simulink model "controled_three_phase_rectifier"  (R2023a)
settings: Solver=ode1be  StartTime=0.0  StopTime=sim_time  FixedStep=50e-6  RelTol=1e-3
values from neighbouring files (symbols this model uses):
  alpha1 = 20    [controled_three_phase_rectifier_script.m]
  alpha2 = 50    [controled_three_phase_rectifier_script.m]
  alpha_steptime1 = 0.4    [controled_three_phase_rectifier_script.m]
  alpha_steptime2 = 0.8    [controled_three_phase_rectifier_script.m]
  gridfreq = 50    [controled_three_phase_rectifier_script.m]
  Rload = 1    [controled_three_phase_rectifier_script.m]
  Vgrid = 6000    [controled_three_phase_rectifier_script.m]
undefined symbols (not defined in the file or in its folder): D1, lagging, pulse
libraries: fl_lib x17, ee_lib x10, nesl_utility x9, batteryecm_lib x1, spsPLL3phLib x1, spsPulseGeneratorThyristor6PulseLib x1
settings Model: Creator=citcea  LastModifiedBy=citcea

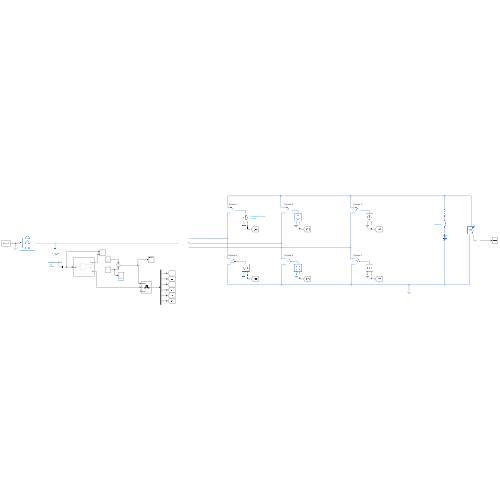
[thumbnail: Simulink's stored preview of the top-level diagram]
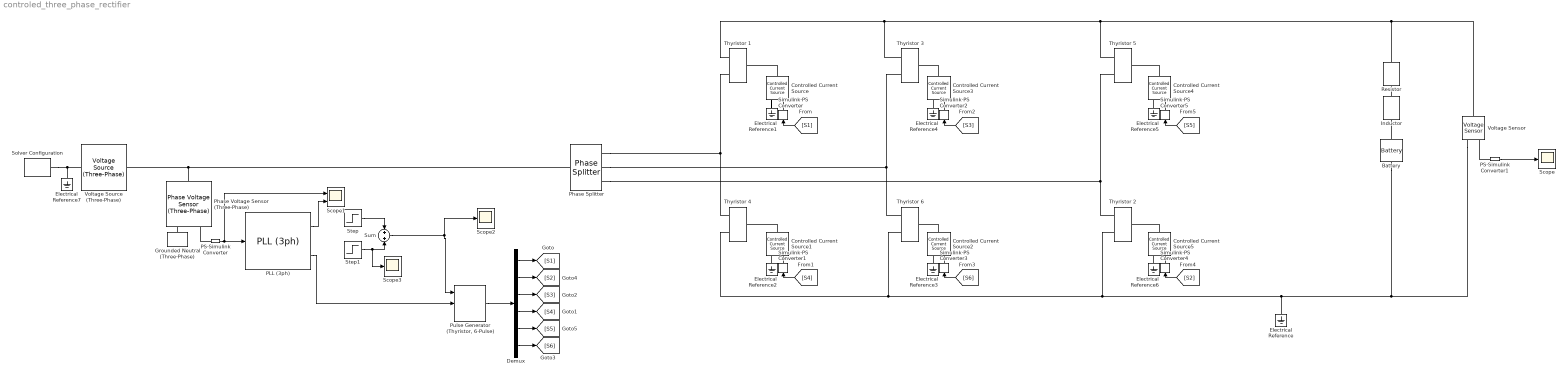
== system controled_three_phase_rectifier ==
  Battery : batteryecm_lib/Battery  Vnom=VDC V  prm_dir=simscape.enum.battery.prm_dir.disabled  R1_dis=2 Ohm  R1_ch=2 Ohm  R1=2 Ohm  prm_AH=simscape.enum.battery.prm_AH.infinite  AH=50 A*hr  V1=11.5 V  AH1=25 A*hr  prm_R2=simscape.enum.battery.prm_R2.disabled  R2=2000 Ohm  Tmeas=298.15 K  charge_measurement_port=simscape.enum.battery.enable.no  prm_dyn=simscape.enum.battery.prm_dyn.off  Rp1=0.005 Ohm  tau1=30 s  Rp2=0.005 Ohm  tau2=30 s  Rp3=0.005 Ohm  tau3=30 s  Rp4=0.005 Ohm  tau4=30 s  Rp5=0.005 Ohm  tau5=30 s  prm_fade=simscape.enum.battery.prm_fade.disabled  N_fade=100  AH_fade=45 A*hr  R1_fade=2.02 Ohm  R1_ch_fade=2.02 Ohm  V1_fade=10.35 V  prm_age=simscape.enum.battery.prm_age.disabled  prm_age_OCV=simscape.enum.battery.prm_age_OCV.OCV  OCV_age=0.9  SOC_age=60  Tmeas_age=298.15 K  delta_time_age_vec=[0] d  temperature_age_vec=[273] K  OCV_scaling_age=2.2134e6  OCV_offset_age=1.632e6  temp_exp_age=0.515833569 V  t_exp_age=0.75  Vnom_T2=12 V  R1_T2=2.2 Ohm  R1_T2_dis=2.2 Ohm  R1_T2_ch=2.2 Ohm  V1_T2=11.4 V  R2_T2=2200 Ohm  Rp1_T2=0.005 Ohm  tau1_T2=30 s  Rp2_T2=0.005 Ohm  tau2_T2=30 s  Rp3_T2=0.005 Ohm  tau3_T2=30 s  Rp4_T2=0.005 Ohm  tau4_T2=30 s  Rp5_T2=0.005 Ohm  tau5_T2=30 s  Tmeas2=273.15 K  thermal_port=simscape.enum.thermaleffects.omit  thermal_mass=30000 J/K  i_specify=off  i_priority=None  i=0 A  i_nominal_specify=off  i_nominal_unit=A  i_nominal_value=1  v_specify=off  v_priority=None  v=0 V  v_nominal_specify=off  v_nominal_unit=V  v_nominal_value=1  charge_specify=off  charge_priority=High  charge=50 A*hr  charge_nominal_specify=off  charge_nominal_unit=A*hr  charge_nominal_value=1  num_cycles_specify=off  num_cycles_priority=High  num_cycles=0  num_cycles_nominal_specify=off  num_cycles_nominal_unit=1  num_cycles_nominal_value=1  temperature_specify=off  temperature_priority=High  temperature=298.15 K  temperature_nominal_specify=off  temperature_nominal_unit=K  temperature_nominal_value=1
  Controlled Current Source{,1..5} (6 alike) : fl_lib/Electrical/Electrical Sources/Controlled Current Source
  Demux : Demux  Outputs=6
  Electrical Reference{,1..7} (8 alike) : fl_lib/Electrical/Electrical Elements/Electrical Reference
  Grounded Neutral (Three-Phase) : ee_lib/Connectors & References/Grounded Neutral (Three-Phase)
  Inductor : fl_lib/Electrical/Electrical Elements/Inductor  l=Lload H  r=0 Ohm  g=1e-9 1/Ohm  i_specify=off  i_priority=None  i=0 A  i_nominal_specify=off  i_nominal_unit=A  i_nominal_value=1  v_specify=off  v_priority=None  v=0 V  v_nominal_specify=off  v_nominal_unit=V  v_nominal_value=1  i_L_specify=off  i_L_priority=High  i_L=0 A  i_L_nominal_specify=off  i_L_nominal_unit=A  i_L_nominal_value=1
  PLL (3ph) : spsPLL3phLib/PLL (3ph)  Fmin=45  Par_Init=[0, gridfreq]  ParK=[180, 3200, 1]  TcD=1e-4  MaxRateChangeFreq=12  FilterCutOffFreq=25  Ts=0  AGC=on
  PS-Simulink Converter : nesl_utility/PS-Simulink Converter  PhysicalDomain=network_engine_domain  SubClassName=ps_output  LeftPortType=input  RightPortType=output  PseudoPeriodic=off  Frequencies=[]  VectorFormat=inherit  Unit=inherit  AffineConversion=off
  PS-Simulink Converter1 : nesl_utility/PS-Simulink Converter  PhysicalDomain=network_engine_domain  SubClassName=ps_output  LeftPortType=input  RightPortType=output  PseudoPeriodic=off  Frequencies=[]  VectorFormat=inherit  Unit=inherit  AffineConversion=off
  Phase Splitter : ee_lib/Connectors & References/Phase Splitter
  Phase Voltage Sensor (Three-Phase) : ee_lib/Sensors & Transducers/Phase Voltage Sensor (Three-Phase)
  "Pulse Generator (Thyristor, 6-Pulse)" : spsPulseGeneratorThyristor6PulseLib/Pulse Generator (Thyristor, 6-Pulse)  GenType=6-pulse  Delta=D1 (lagging)  pwidth=60  Double_Pulse=off  Ts=0
      settings: LibrarySourceBlock=|
      | sps_lib/Power Electronics/Power Electronics Control/Pulse Generator
      | (Thyristor, 6-Pulse)
  Resistor : fl_lib/Electrical/Electrical Elements/Resistor  R=Rload Ohm  i_specify=off  i_priority=None  i=0 A  i_nominal_specify=off  i_nominal_unit=A  i_nominal_value=1  v_specify=off  v_priority=None  v=0 V  v_nominal_specify=off  v_nominal_unit=V  v_nominal_value=1
  Scope : Scope
  Scope1 : Scope  NumInputPorts=2
  Scope2 : Scope
  Scope3 : Scope
  Simulink-PS Converter{,1..5} (6 alike) : nesl_utility/Simulink-PS Converter  PhysicalDomain=network_engine_domain  SubClassName=ps_input  LeftPortType=input  RightPortType=output  PseudoPeriodic=off  Frequencies=[]  NoiseDistribution=none  NoiseParameters=[]  Unit=1  AffineConversion=off  FilteringAndDerivatives=provide  SimscapeFilterOrder=1  InputFilterTimeConstant=0.001  UdotUserProvided=0
  Solver Configuration : nesl_utility/Solver Configuration  PhysicalDomain=network_engine_domain  SubClassName=solver  LeftPortType=input  RightPortType=generic  Tones=[]  Harmonics=[]  SimulateNoise=off  Profile=off  UseLocalSampling=off  EnableSwitchedLinearOptims=on  FrequencyDomain=off  UseCCode=off  RelTol=0.001  AbsTol=0.001  MinStep=1e-09  ToWorkspace=off  RevertToSquareIcSolve=off  NumHomotopyIterations=100  PhasorMode=off  PhasorModeNumHarmonics=1  ConsistencySolver=NEWTON_XTOL_AFTER_FTOL  IndexReductionMethod=DerivativeReplacement  DoDC=off  ResidualTolerance=1e-09  ConsistencyTolSource=GLOBAL  ConsistencyAbsTol=0.001  ConsistencyRelTol=0.001  ConsistencyTolFactor=0.001  UseLocalSolver=on  LocalSolverChoice=NE_BACKWARD_EULER_ADVANCER  ResolveIndetEquations=on  FunctionEvalNumThread=1  LocalSolverSampleTime=50e-6  DoFixedCost=on  MaxNonlinIter=3  MaxModeIter=2  ComputeImpulses=off  ImpulseIterations=2  LinearAlgebra=auto  LinearAlgebraNumThread=0  EquationFormulation=NE_TIME_EF  DelaysMemoryBudget=1024  AutomaticFiltering=on  FilteringTimeConstant=0.001  PartitionStorageMethod=AS_NEEDED  PartitionMemoryBudget=1024  PartitionMethod=ROBUST
  Step : Step  Time=alpha_steptime1  After=alpha1  SampleTime=0
  Step1 : Step  Time=alpha2-alpha1  After=alpha_steptime2  SampleTime=0
  Sum : Sum
  Thyristor {1..3,5..6} (5 alike) : ee_lib/Semiconductors & Converters/Thyristor  model_type=ee.enum.semiconductors.thyristorModelType.equations  v_on=1.2 V  i_on=1 A  VT_vec=[.75, 1, 1.25, 1.5, 1.75, 2, 2.25] V  IT_vec=[.015, .22, .75, 1.4, 2, 2.75, 3.45] A  IDRM=0.01 mA  VDRM=400 V  i_H=1 mA  Tmeas=25 degC  i_GT=3 uA  v_GT=0.6 V  V_D=12 V  R=120 Ohm  dVdt=150 V/us  R_GK=1000 Ohm  TF_NPN_parameterization=1  T_d=2 us  i_d=10 mA  TF_NPN=0.3 us  TF_PNP_parameterization=1  TF_PNP=0.3 us  t_on_delay=0 s  t_on_curr=1 mA  t_on_rise=0 s  Rs=87 kOhm  Rgate=10 Ohm  Gain=10  ig_specify=off  ig_priority=None  ig=0 A  ig_nominal_specify=off  ig_nominal_unit=A  ig_nominal_value=1  ia_specify=off  ia_priority=None  ia=0 A  ia_nominal_specify=off  ia_nominal_unit=A  ia_nominal_value=1  vgk_specify=off  vgk_priority=None  vgk=0 V  vgk_nominal_specify=off  vgk_nominal_unit=V  vgk_nominal_value=1  vak_specify=off  vak_priority=None  vak=0 V  vak_nominal_specify=off  vak_nominal_unit=V  vak_nominal_value=1  v_npn_Cbc_specify=off  v_npn_Cbc_priority=High  v_npn_Cbc=0 V  v_npn_Cbc_nominal_specify=off  v_npn_Cbc_nominal_unit=V  v_npn_Cbc_nominal_value=1  v_npn_Cbe_specify=off  v_npn_Cbe_priority=High  v_npn_Cbe=0 V  v_npn_Cbe_nominal_specify=off  v_npn_Cbe_nominal_unit=V  v_npn_Cbe_nominal_value=1  v_pnp_Cbe_specify=off  v_pnp_Cbe_priority=High  v_pnp_Cbe=0 V  v_pnp_Cbe_nominal_specify=off  v_pnp_Cbe_nominal_unit=V  v_pnp_Cbe_nominal_value=1  thermal_network_parameterization=ee.enum.thermalNetworkTopology.junctionCase  Rth=[0, 10] K/W  Rth_Cauer=[1, 3, 10] K/W  Rth_Foster=[4, 6] K/W  thermal_mass_parameterization=ee.enum.thermalNetwork.timeconstant  thermal_mass=[0, 1] J/K  thermal_mass_Cauer=[.1, .3, 1] J/K  thermal_mass_Foster=[1.5, 3] J/K  thermal_time_constant=[0, 10] s  thermal_time_constant_Cauer=[1, 3, 10] s  thermal_time_constant_Foster=[6, 18] s  thermal_mass_initial_temperatures=[25, 25] degC  thermal_mass_initial_temperatures_Cauer=[25, 25, 25] degC  Tvec_initial_Foster=[25, 25, 25, 25] degC
      settings: InternalSimscapePortConfiguration="{\"Bottom\":[],\"Left\":[{\"id\":\"G\",\"label\":\"\",\"type\":\"foundation.electrical.electrical\"}],\"Right\":[{\"id\":\"A\",\"label\":\"\",\"type\":\"foundation.electrical.electrical\"},{\"id\":\"K\",\"label\":\"\",\"type\":\"foundation.electrical.electrical\"}],\"Top\":[]}"
  "Thyristor 4 " : ee_lib/Semiconductors & Converters/Thyristor  model_type=ee.enum.semiconductors.thyristorModelType.equations  v_on=1.2 V  i_on=1 A  VT_vec=[.75, 1, 1.25, 1.5, 1.75, 2, 2.25] V  IT_vec=[.015, .22, .75, 1.4, 2, 2.75, 3.45] A  IDRM=0.01 mA  VDRM=400 V  i_H=1 mA  Tmeas=25 degC  i_GT=3 uA  v_GT=0.6 V  V_D=12 V  R=120 Ohm  dVdt=150 V/us  R_GK=1000 Ohm  TF_NPN_parameterization=1  T_d=2 us  i_d=10 mA  TF_NPN=0.3 us  TF_PNP_parameterization=1  TF_PNP=0.3 us  t_on_delay=0 s  t_on_curr=1 mA  t_on_rise=0 s  Rs=87 kOhm  Rgate=10 Ohm  Gain=10  ig_specify=off  ig_priority=None  ig=0 A  ig_nominal_specify=off  ig_nominal_unit=A  ig_nominal_value=1  ia_specify=off  ia_priority=None  ia=0 A  ia_nominal_specify=off  ia_nominal_unit=A  ia_nominal_value=1  vgk_specify=off  vgk_priority=None  vgk=0 V  vgk_nominal_specify=off  vgk_nominal_unit=V  vgk_nominal_value=1  vak_specify=off  vak_priority=None  vak=0 V  vak_nominal_specify=off  vak_nominal_unit=V  vak_nominal_value=1  v_npn_Cbc_specify=off  v_npn_Cbc_priority=High  v_npn_Cbc=0 V  v_npn_Cbc_nominal_specify=off  v_npn_Cbc_nominal_unit=V  v_npn_Cbc_nominal_value=1  v_npn_Cbe_specify=off  v_npn_Cbe_priority=High  v_npn_Cbe=0 V  v_npn_Cbe_nominal_specify=off  v_npn_Cbe_nominal_unit=V  v_npn_Cbe_nominal_value=1  v_pnp_Cbe_specify=off  v_pnp_Cbe_priority=High  v_pnp_Cbe=0 V  v_pnp_Cbe_nominal_specify=off  v_pnp_Cbe_nominal_unit=V  v_pnp_Cbe_nominal_value=1  thermal_network_parameterization=ee.enum.thermalNetworkTopology.junctionCase  Rth=[0, 10] K/W  Rth_Cauer=[1, 3, 10] K/W  Rth_Foster=[4, 6] K/W  thermal_mass_parameterization=ee.enum.thermalNetwork.timeconstant  thermal_mass=[0, 1] J/K  thermal_mass_Cauer=[.1, .3, 1] J/K  thermal_mass_Foster=[1.5, 3] J/K  thermal_time_constant=[0, 10] s  thermal_time_constant_Cauer=[1, 3, 10] s  thermal_time_constant_Foster=[6, 18] s  thermal_mass_initial_temperatures=[25, 25] degC  thermal_mass_initial_temperatures_Cauer=[25, 25, 25] degC  Tvec_initial_Foster=[25, 25, 25, 25] degC
      settings: InternalSimscapePortConfiguration="{\"Bottom\":[],\"Left\":[{\"id\":\"G\",\"label\":\"\",\"type\":\"foundation.electrical.electrical\"}],\"Right\":[{\"id\":\"A\",\"label\":\"\",\"type\":\"foundation.electrical.electrical\"},{\"id\":\"K\",\"label\":\"\",\"type\":\"foundation.electrical.electrical\"}],\"Top\":[]}"
  Voltage Source (Three-Phase) : ee_lib/Sources/Voltage Source (Three-Phase)  vline_rms=sqrt(3) * Vgrid V  shift=0 deg  freq=gridfreq Hz  impedance_option=0  SShortCircuit=1e6 A*V  XR=15  R=0.01 Ohm  L=3.97e-4 H  harmonic_option=0  harmonic_orders=[5, 7, 11, 13]  harmonic_ratios=[.1, .1, .1, .1]  G_parasitic=0 1/Ohm  I_specify=off  I_priority=None  I=[0, 0, 0] A  I_nominal_specify=off  I_nominal_unit=A  I_nominal_value=1
  Voltage Sensor : fl_lib/Electrical/Electrical Sensors/Voltage Sensor
  wires:
  [S1] -> Simulink-PS Converter/1
  [S4] -> Simulink-PS Converter1/1
  [S3] -> Simulink-PS Converter2/1
  [S6] -> Simulink-PS Converter3/1
  [S2] -> Simulink-PS Converter4/1
  [S5] -> Simulink-PS Converter5/1
  PS-Simulink Converter/1 -> Scope1/1, PLL (3ph)/1
  PLL (3ph)/2 -> "Pulse Generator (Thyristor, 6-Pulse)"/2
  "Pulse Generator (Thyristor, 6-Pulse)"/1 -> Demux/1
  Demux/1 -> [S1]
  Demux/2 -> [S2]
  Demux/3 -> [S3]
  Demux/4 -> [S4]
  Demux/6 -> [S6]
  Demux/5 -> [S5]
  PLL (3ph)/1 -> Scope1/2
  PS-Simulink Converter1/1 -> Scope/1
  Sum/1 -> "Pulse Generator (Thyristor, 6-Pulse)"/1, Scope2/1
  Step/1 -> Sum/1
  Step1/1 -> Scope3/1, Sum/2
  connections:
  "Thyristor 4 "/RConn2 -- Phase Splitter/RConn1 -- Thyristor 1/RConn1
  Thyristor 6/RConn2 -- Phase Splitter/RConn2 -- Thyristor 3/RConn1
  Thyristor 2/RConn2 -- Phase Splitter/RConn3 -- Thyristor 5/RConn1
  Thyristor 2/RConn1 -- Voltage Sensor/RConn2 -- Battery/RConn1 -- Electrical Reference/LConn1 -- Thyristor 6/RConn1 -- "Thyristor 4 "/RConn1
  Thyristor 5/RConn2 -- Voltage Sensor/LConn1 -- Resistor/LConn1 -- Thyristor 3/RConn2 -- Thyristor 1/RConn2
  Battery/LConn1 -- Inductor/RConn1
  Inductor/LConn1 -- Resistor/RConn1
  Controlled Current Source/LConn1 -- Thyristor 1/LConn1
  Electrical Reference1/LConn1 -- Controlled Current Source/RConn2
  Electrical Reference2/LConn1 -- Controlled Current Source1/RConn2
  Controlled Current Source1/LConn1 -- "Thyristor 4 "/LConn1
  Electrical Reference3/LConn1 -- Controlled Current Source2/RConn2
  Controlled Current Source2/LConn1 -- Thyristor 6/LConn1
  Electrical Reference4/LConn1 -- Controlled Current Source3/RConn2
  Controlled Current Source3/LConn1 -- Thyristor 3/LConn1
  Electrical Reference5/LConn1 -- Controlled Current Source4/RConn2
  Controlled Current Source4/LConn1 -- Thyristor 5/LConn1
  Electrical Reference6/LConn1 -- Controlled Current Source5/RConn2
  Controlled Current Source5/LConn1 -- Thyristor 2/LConn1
  Simulink-PS Converter/RConn1 -- Controlled Current Source/RConn1
  Simulink-PS Converter1/RConn1 -- Controlled Current Source1/RConn1
  Simulink-PS Converter2/RConn1 -- Controlled Current Source3/RConn1
  Simulink-PS Converter3/RConn1 -- Controlled Current Source2/RConn1
  Simulink-PS Converter4/RConn1 -- Controlled Current Source5/RConn1
  Simulink-PS Converter5/RConn1 -- Controlled Current Source4/RConn1
  Phase Voltage Sensor (Three-Phase)/LConn1 -- Phase Splitter/LConn1 -- Voltage Source (Three-Phase)/RConn1
  Solver Configuration/RConn1 -- Electrical Reference7/LConn1 -- Voltage Source (Three-Phase)/LConn1
  Grounded Neutral (Three-Phase)/LConn1 -- Phase Voltage Sensor (Three-Phase)/RConn2
  PS-Simulink Converter/LConn1 -- Phase Voltage Sensor (Three-Phase)/RConn1
  PS-Simulink Converter1/LConn1 -- Voltage Sensor/RConn1
